simulink model "CraneStab"  (Simulink 8.6)
settings: Solver=ode1  SolverMode=SingleTasking  StartTime=0.0  StopTime=40  FixedStep=0.001  RelTol=1e-3
undefined symbols (not defined in the file): Advantech, PCI
libraries: sldrtlib x11
settings Model: Creator=Demo11  LastModifiedBy=demo  SimulationMode=external  ExtModeTrigMode=oneshot  ExtModeTrigDuration=100000
settings DataIOCC: LimitDataPoints=off  SignalLoggingName=sigsOut
settings OptimizationCC: BlockReduction=off  BooleanDataType=off  InitFltsAndDblsToZero=on
settings DebuggingCC: SaveWithParameterizedLinksMsg=none  SignalResolutionControl=TryResolveAllWithWarning  SolverPrmCheckMsg=none  MultiTaskDSMMsg=warning  MultiTaskCondExecSysMsg=none  FcnCallInpInsideContextMsg=UseLocalSettings
settings HardwareCC: ProdBitPerLong=64  ProdBitPerPointer=64  ProdIntDivRoundTo=Zero  ProdEndianess=LittleEndian  ProdWordSize=64  ProdHWDeviceType=Intel->x86-64  TargetBitPerLong=64  TargetBitPerPointer=64  TargetIntDivRoundTo=Zero  TargetEndianess=LittleEndian  TargetWordSize=64  TargetHWDeviceType=Intel->x86-64
settings RTWCC: SystemTargetFile=sldrt.tlc  TemplateMakefile=sldrt.tmf  Description=Simulink Desktop Real-Time  RTWCompilerOptimization=on
settings CodeAppCC: MaxIdLength=95
settings SimulinkDesktopRealTimeCC: TargetPreCompLibLocation=C:\Program Files\MATLAB\R2015b\toolbox\sldrt\lib\win64  TargetLangStandard=C89/C90 (ANSI)  SupportVariableSizeSignals=off

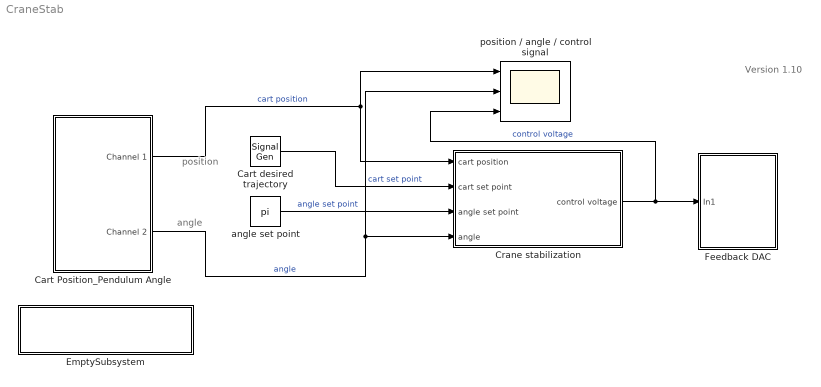
== system CraneStab ==
  note: position
  note: angle
  note: Version 1.10
  Cart Position_Pendulum Angle : Subsystem  mask(Feedback Encoder Block){st=0.001, of1=0, of2=-1024}
      mask prompts: st "Sample Time"; of1 "Channel 1 Offset"; of2 "Channel 2 Offset"
      mask help: Special block to use with the Feedback experiments to read encoder channels using the digital I/O lines
      mask Display:
      | image(imread('bckg.bmp'))
      | disp('PCI1711 \n Lab I/O Board \n\n\n Feedback Encoder')
  "Cart desired trajectory " : SignalGenerator  Amplitude=0.3  Frequency=0.1
  Crane stabilization : Subsystem
      mask Display:
      | image(imread('bckg.bmp'))
      | disp('Crane stabilization')
  EmptySubsystem : Subsystem
      mask Display:
      | image(imread('FB-inst-blue2.jpg'))
      | disp('\n\nFeedback Instruments Limited')
  Feedback DAC : Subsystem  mask(DAC Unit for Feedback Experiments){st=0.001, ch=1}
      mask prompts: st "Sample Time"; ch "Output Channel"
      mask help:
      | Digital to Analog Output  for Feedback Experiments
      | using Advantech PCI1711  I/O board
      mask Display:
      | image(imread('bckg.bmp'))
      | disp('PCI1711 \n Lab I/O Board \n\n Feedback  DAC')
  angle set point : Constant  Value=pi
  position / angle / control signal : Scope  NumInputPorts=3
      mask Display: image(imread('scope.jpg'))
  wires:
  Crane stabilization/1(control voltage) -> Feedback DAC/1(In1), position / angle / control signal/3  "control voltage"
  angle set point/1 -> Crane stabilization/3(angle set point)  "angle set point"
  Cart Position_Pendulum Angle/2(Channel 2) -> Crane stabilization/4(angle), position / angle / control signal/2  "angle"
  Cart Position_Pendulum Angle/1(Channel 1) -> Crane stabilization/1(cart position), position / angle / control signal/1  "cart position"
  "Cart desired trajectory "/1 -> Crane stabilization/2(cart set point)  "cart set point"

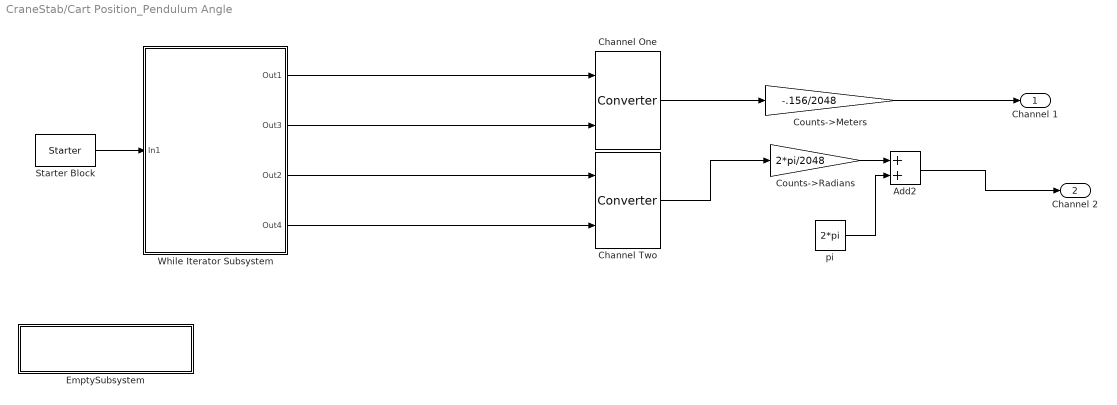
== system CraneStab/Cart Position_Pendulum Angle ==
  Add2 : Sum
  Channel One : S-Function  FunctionName=Converter  Parameters=of1,st  SFunctionDeploymentMode=off  EnableBusSupport=off
  Channel Two : S-Function  FunctionName=Converter  Parameters=of2,st  SFunctionDeploymentMode=off  EnableBusSupport=off
  Counts->Meters : Gain  Gain=-.156/2048  SaturateOnIntegerOverflow=on  OutDataTypeStr=Inherit: Same as input  ParamDataTypeStr=Inherit: Same as input
  Counts->Radians : Gain  Gain=2*pi/2048  SaturateOnIntegerOverflow=on  OutDataTypeStr=Inherit: Same as input  ParamDataTypeStr=Inherit: Same as input
  EmptySubsystem : Subsystem
      mask Display:
      | image(imread('FB-inst-blue2.jpg'))
      | disp('\n\nFeedback Instruments Limited')
  Starter Block : S-Function  FunctionName=Starter  Parameters=sample_time  SFunctionDeploymentMode=off  EnableBusSupport=off  mask{sample_time=st}
      mask prompts: sample_time "Sample Time:"
  While Iterator Subsystem : Subsystem  TreatAsAtomicUnit=on
  pi : Constant  Value=2*pi
  Channel 1 : Outport
  Channel 2 : Outport  Port=2
  wires:
  Add2/1 -> Channel 2/1
  Channel Two/1 -> Counts->Radians/1
  pi/1 -> Add2/2
  Counts->Radians/1 -> Add2/1
  Counts->Meters/1 -> Channel 1/1
  Starter Block/1 -> While Iterator Subsystem/1(In1)
  While Iterator Subsystem/1(Out1) -> Channel One/1
  While Iterator Subsystem/2(Out3) -> Channel One/2
  While Iterator Subsystem/3(Out2) -> Channel Two/1
  While Iterator Subsystem/4(Out4) -> Channel Two/2
  Channel One/1 -> Counts->Meters/1

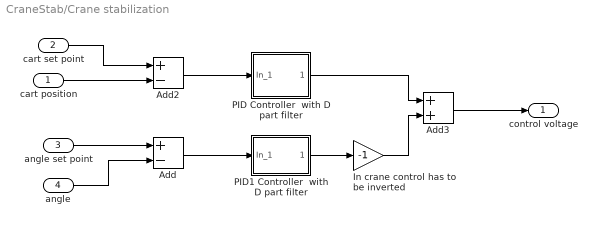
== system CraneStab/Crane stabilization ==
  cart position : Inport
  cart set point : Inport  Port=2
  angle set point : Inport  Port=3
  angle : Inport  Port=4
  Add : Sum  Inputs=+-
  Add2 : Sum  Inputs=+-
  Add3 : Sum
  In crane control has to be inverted : Gain  Gain=-1
  PID Controller  with D part filter : Subsystem  AncestorBlock=simulink_extras/Additional Linear/PID Controller  mask(PID Controller){P=8, I=0.3, D=4}
      mask prompts: P "Proportional:"; I "Integral:"; D "Derivative:"
      mask help:
      | Enter expressions for proportional, integral, and derivative terms.
      | P+I/s+Ds
      mask Help: This block implements a PID controller where parameters are entered for the Proportional, Integral and Derivative terms. Unmask this block to see how it works. The derivative term is implemented using a true derivative block.
      mask Callback P:
      | if str2num(get_param(gcb, 'P'))>12
      |  WARNDLG('Proportional Gain is out of the range [4..12] and is set to maximum value now', 'Setting Value Error')
      |  set_param(gcb,'P','12');
      | end
      | if str2num(get_param(gcb, 'P'))<4
      |  WARNDLG('Proportional Gain is out of the range [4..12] and is set to minimum now', 'Setting Value Error')
      |  set_param(gcb,'P','4');
      | end
      mask Callback I:
      | if str2num(get_param(gcb, 'I'))>0.5
      |  WARNDLG('Integral Gain is out of the range [0.1 .. 0.5] and is set to maximum value now', 'Setting Value Error')
      |  set_param(gcb,'I','0.5');
      | end
      | if str2num(get_param(gcb, 'I'))<0.1
      |  WARNDLG('Integral Gain is out of the range [0.1 .. 0.5] and is set to minimum now', 'Setting Value Error')
      |  set_param(gcb,'I','0.1');
      | end
      mask Callback D:
      | if str2num(get_param(gcb, 'D'))>6
      |  WARNDLG('Derivative Gain is out of the range [2..6] and is set to maximum value now', 'Setting Value Error')
      |  set_param(gcb,'D','6');
      | end
      | if str2num(get_param(gcb, 'D'))<2
      |  WARNDLG('Derivative Gain is out of the range [2..6] and is set to minimum now', 'Setting Value Error')
      |  set_param(gcb,'D','2');
      | end
      mask Display:
      | image(imread('bckg.bmp'))
      | disp('PID')
  PID1 Controller  with D part filter : Subsystem  AncestorBlock=simulink_extras/Additional Linear/PID Controller  mask(PID Controller){P=5, I=0.1, D=0.2}
      mask prompts: P "Proportional:"; I "Integral:"; D "Derivative:"
      mask help:
      | Enter expressions for proportional, integral, and derivative terms.
      | P+I/s+Ds
      mask Help: This block implements a PID controller where parameters are entered for the Proportional, Integral and Derivative terms. Unmask this block to see how it works. The derivative term is implemented using a true derivative block.
      mask Callback P:
      | if str2num(get_param(gcb, 'P'))>8
      |  WARNDLG('Proportional Gain is out of the range [2..8] and is set to maximum value now', 'Setting Value Error')
      |  set_param(gcb,'P','8');
      | end
      | if str2num(get_param(gcb, 'P'))<2
      |  WARNDLG('Proportional Gain is out of the range [2..8] and is set to minimum now', 'Setting Value Error')
      |  set_param(gcb,'P','2');
      | end
      mask Callback I:
      | if str2num(get_param(gcb, 'I'))>0.15
      |  WARNDLG('Integral Gain is out of the range [0.05 .. 0.15] and is set to maximum value now', 'Setting Value Error')
      |  set_param(gcb,'I','0.15');
      | end
      | if str2num(get_param(gcb, 'I'))<0.05
      |  WARNDLG('Integral Gain is out of the range [0.05 .. 0.15] and is set to minimum now', 'Setting Value Error')
      |  set_param(gcb,'I','0.05');
      | end
      mask Callback D:
      | if str2num(get_param(gcb, 'D'))>0.3
      |  WARNDLG('Derivative Gain is out of the range [0.1 .. 0.3] and is set to maximum value now', 'Setting Value Error')
      |  set_param(gcb,'D','0.3');
      | end
      | if str2num(get_param(gcb, 'D'))<0.1
      |  WARNDLG('Derivative Gain is out of the range [0.1 .. 0.3] and is set to minimum now', 'Setting Value Error')
      |  set_param(gcb,'D','0.1');
      | end
      mask Display:
      | image(imread('bckg.bmp'))
      | disp('PID')
  control voltage : Outport
  wires:
  angle/1 -> Add/2
  angle set point/1 -> Add/1
  cart set point/1 -> Add2/1
  cart position/1 -> Add2/2
  Add3/1 -> control voltage/1
  PID Controller  with D part filter/1(Out_1) -> Add3/1
  Add2/1 -> PID Controller  with D part filter/1(In_1)
  Add/1 -> PID1 Controller  with D part filter/1(In_1)
  In crane control has to be inverted/1 -> Add3/2
  PID1 Controller  with D part filter/1(Out_1) -> In crane control has to be inverted/1

== system CraneStab/EmptySubsystem ==

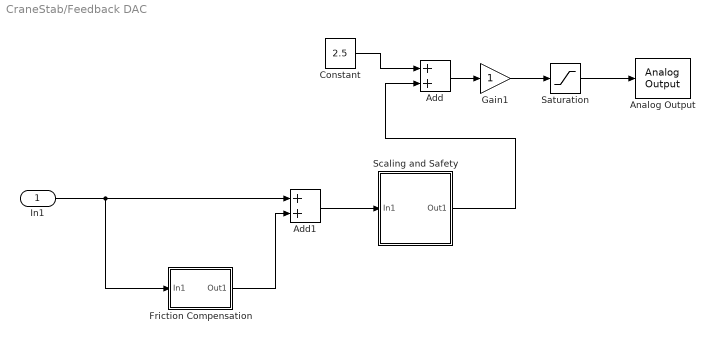
== system CraneStab/Feedback DAC ==
  In1 : Inport
  Add : Sum  OutDataTypeStr=Inherit: Same as first input
  Add1 : Sum
  Analog Output : sldrtlib/Analog Output  SampleTime=st  MaxMissedTicks=10  ShowMissedTicks=off  YieldWhenWaiting=off  DrvName=Advantech/PCI-1711  DrvAddress=4294967295  DrvOptions=zeros(1,0)  Channels=ch  RangeMode=1  VoltRange=2  InitialValue=2.5  FinalValue=2.5
      settings: AttributesFormatString=Advantech\nPCI-1711 [auto]
  Constant : Constant  Value=2.5
  Friction Compensation : Subsystem  mask(linear){frictionCompNeg=.1, frictionCompPos=.1}
      mask prompts: frictionCompNeg "Friction Compensation Magnitude in Negative Direction"; frictionCompPos "Friction Compensation Magnitude in Positive Direction"
      mask Display: plot(0,0,100,100,[40,30,20],[87,85,80],[46,54,54,46,46],[90,90,80,80,90],[46,45,45,46,54,55,55,54,46],[78,80,90,91,91,90,80,78,78],[51,51,49,49],[78,10,10,78],[90,80,70,60],[70,80,85,88],[20,10],[80,70],[20,20,15],[73,80,80],[85,80,80],[80,80,74])
  Gain1 : Gain
  Saturation : Saturate  UpperLimit=5.0  LowerLimit=0
  Scaling and Safety : Subsystem
  wires:
  Add1/1 -> Scaling and Safety/1(In1)
  In1/1 -> Add1/1, Friction Compensation/1(In1)
  Friction Compensation/1(Out1) -> Add1/2
  Constant/1 -> Add/1
  Saturation/1 -> Analog Output/1
  Add/1 -> Gain1/1
  Gain1/1 -> Saturation/1
  Scaling and Safety/1(Out1) -> Add/2

== system CraneStab/Cart Position_Pendulum Angle/EmptySubsystem ==

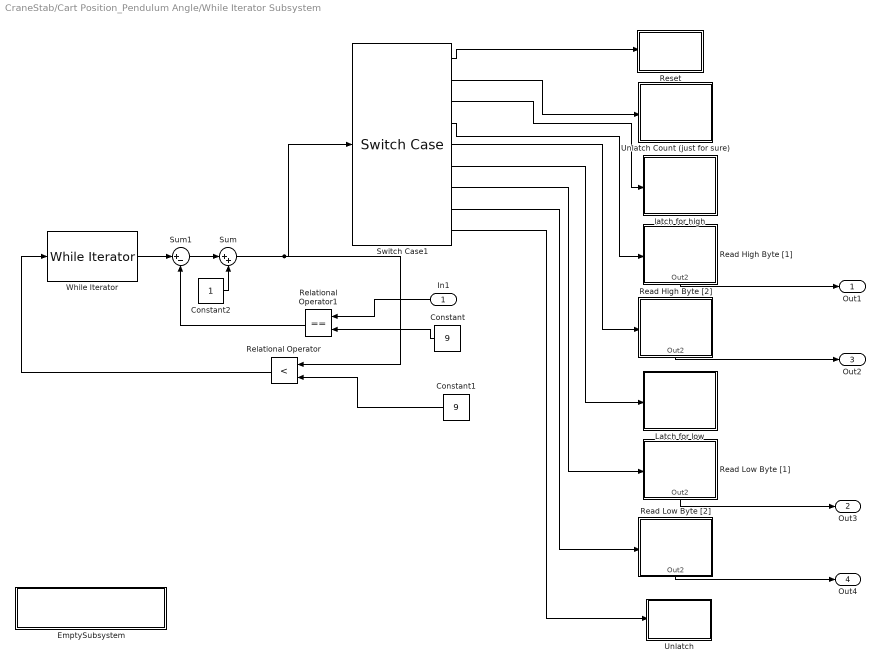
== system CraneStab/Cart Position_Pendulum Angle/While Iterator Subsystem ==
  In1 : Inport
  Constant : Constant  Value=9
  Constant1 : Constant  Value=9
  Constant2 : Constant
  EmptySubsystem : Subsystem
      mask Display:
      | image(imread('FB-inst-blue2.jpg'))
      | disp('\n\nFeedback Instruments Limited')
  Latch for low : Subsystem  TreatAsAtomicUnit=on
  Read High Byte [1] : Subsystem  TreatAsAtomicUnit=on
  Read High Byte [2] : Subsystem  TreatAsAtomicUnit=on
  Read Low Byte [1] : Subsystem  TreatAsAtomicUnit=on
  Read Low Byte [2] : Subsystem  TreatAsAtomicUnit=on
  Relational Operator : RelationalOperator  Operator=<  OutDataTypeStr=boolean
  Relational Operator1 : RelationalOperator  Operator===  OutDataTypeStr=boolean
  Reset : Subsystem  TreatAsAtomicUnit=on
  Sum : Sum  Inputs=|++
  Sum1 : Sum  Inputs=|+-  OutDataTypeStr=Inherit: Same as first input
  Switch Case1 : SwitchCase  CaseConditions={1,2,3,4,5,6,7,8,9}  ShowDefaultCase=off
  Unlatch : Subsystem  TreatAsAtomicUnit=on
  "Unlatch Count (just for sure) " : Subsystem  TreatAsAtomicUnit=on
  While Iterator : WhileIterator  MaxIters=9  WhileBlockType=do-while  ResetStates=reset  ShowIterationPort=on  OutputDataType=int8
  latch for high : Subsystem  TreatAsAtomicUnit=on
  Out1 : Outport
  Out3 : Outport  Port=2
  Out2 : Outport  Port=3
  Out4 : Outport  Port=4
  wires:
  Relational Operator/1 -> While Iterator/1
  In1/1 -> Relational Operator1/1
  Constant/1 -> Relational Operator1/2
  Relational Operator1/1 -> Sum1/2
  While Iterator/1 -> Sum1/1
  Switch Case1/1 -> Reset/Action
  Switch Case1/2 -> "Unlatch Count (just for sure) "/Action
  Constant1/1 -> Relational Operator/2
  Read High Byte [1]/1(Out2) -> Out1/1
  Read High Byte [2]/1(Out2) -> Out2/1
  Read Low Byte [1]/1(Out2) -> Out3/1
  Read Low Byte [2]/1(Out2) -> Out4/1
  Sum1/1 -> Sum/1
  Sum/1 -> Switch Case1/1, Relational Operator/1
  Constant2/1 -> Sum/2
  Switch Case1/3 -> latch for high/Action
  Switch Case1/4 -> Read High Byte [1]/Action
  Switch Case1/5 -> Read High Byte [2]/Action
  Switch Case1/6 -> Latch for low/Action
  Switch Case1/7 -> Read Low Byte [1]/Action
  Switch Case1/8 -> Read Low Byte [2]/Action
  Switch Case1/9 -> Unlatch/Action

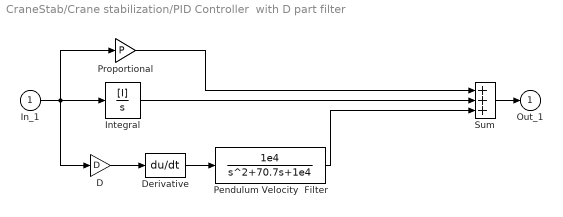
== system CraneStab/Crane stabilization/PID Controller  with D part filter ==
  In_1 : Inport
  D : Gain  Gain=D  SaturateOnIntegerOverflow=on  OutDataTypeStr=Inherit: Same as input  ParamDataTypeStr=Inherit: Same as input
  Derivative : Derivative
  Integral : TransferFcn  Numerator=[I]  Denominator=[1 0]
  Pendulum Velocity  Filter : TransferFcn  Numerator=[1e4]  Denominator=[1 70.7 1e4]
  Proportional : Gain  Gain=P  SaturateOnIntegerOverflow=on  OutDataTypeStr=Inherit: Same as input  ParamDataTypeStr=Inherit: Same as input
  Sum : Sum  Inputs=+++  SaturateOnIntegerOverflow=on  InputSameDT=on  OutDataTypeStr=Inherit: Same as first input
  Out_1 : Outport  InitialOutput=0
  wires:
  Pendulum Velocity  Filter/1 -> Sum/3
  D/1 -> Derivative/1
  Sum/1 -> Out_1/1
  In_1/1 -> Proportional/1, Integral/1, D/1
  Derivative/1 -> Pendulum Velocity  Filter/1
  Integral/1 -> Sum/2
  Proportional/1 -> Sum/1

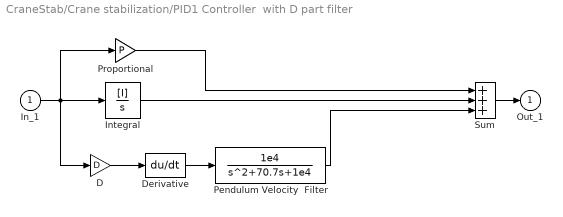
== system CraneStab/Crane stabilization/PID1 Controller  with D part filter ==
  In_1 : Inport
  D : Gain  Gain=D  SaturateOnIntegerOverflow=on  OutDataTypeStr=Inherit: Same as input  ParamDataTypeStr=Inherit: Same as input
  Derivative : Derivative
  Integral : TransferFcn  Numerator=[I]  Denominator=[1 0]
  Pendulum Velocity  Filter : TransferFcn  Numerator=[1e4]  Denominator=[1 70.7 1e4]
  Proportional : Gain  Gain=P  SaturateOnIntegerOverflow=on  OutDataTypeStr=Inherit: Same as input  ParamDataTypeStr=Inherit: Same as input
  Sum : Sum  Inputs=+++  SaturateOnIntegerOverflow=on  InputSameDT=on  OutDataTypeStr=Inherit: Same as first input
  Out_1 : Outport  InitialOutput=0
  wires:
  Proportional/1 -> Sum/1
  Integral/1 -> Sum/2
  Derivative/1 -> Pendulum Velocity  Filter/1
  In_1/1 -> Integral/1, Proportional/1, D/1
  Sum/1 -> Out_1/1
  D/1 -> Derivative/1
  Pendulum Velocity  Filter/1 -> Sum/3

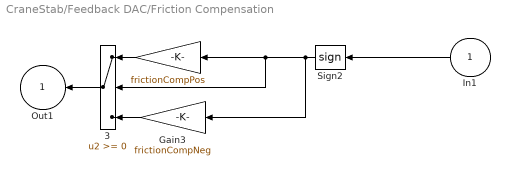
== system CraneStab/Feedback DAC/Friction Compensation ==
  In1 : Inport
  " " : Gain  Gain=frictionCompPos  SaturateOnIntegerOverflow=on  OutDataTypeStr=Inherit: Same as input  ParamDataTypeStr=Inherit: Same as input
  3 : Switch  SaturateOnIntegerOverflow=on  InputSameDT=on
  Gain3 : Gain  Gain=frictionCompNeg  SaturateOnIntegerOverflow=on  OutDataTypeStr=Inherit: Same as input  ParamDataTypeStr=Inherit: Same as input
  Sign2 : Signum  Tag=T
  Out1 : Outport  InitialOutput=0
  wires:
  3/1 -> Out1/1
  Sign2/1 -> 3/2, " "/1, Gain3/1
  Gain3/1 -> 3/3
  " "/1 -> 3/1
  In1/1 -> Sign2/1

== system CraneStab/Feedback DAC/Scaling and Safety ==
  In1 : Inport
  -1 : Gain  Gain=-1  SaturateOnIntegerOverflow=on  OutDataTypeStr=Inherit: Same as input  ParamDataTypeStr=Inherit: Same as input
  Saturation : Saturate  UpperLimit=2.5  LowerLimit=-2.5
  Out1 : Outport
  wires:
  -1/1 -> Saturation/1  "actual LoadPosition"
  In1/1 -> -1/1
  Saturation/1 -> Out1/1

== system CraneStab/Cart Position_Pendulum Angle/While Iterator Subsystem/EmptySubsystem ==

== system CraneStab/Cart Position_Pendulum Angle/While Iterator Subsystem/Latch for low ==
  Action Port : ActionPort  ActionType=case
  Constant : Constant  Value=6  OutDataTypeStr=double
  Digital Output : sldrtlib/Digital Output  SampleTime=-1  MaxMissedTicks=10  ShowMissedTicks=off  YieldWhenWaiting=off  DrvName=Advantech/PCI-1711  DrvAddress=4294967295  DrvOptions=zeros(1,0)  Channels=1  BitMode=2  InitialValue=0  FinalValue=0
      settings: AttributesFormatString=Advantech\nPCI-1711 [auto]
  wires:
  Constant/1 -> Digital Output/1

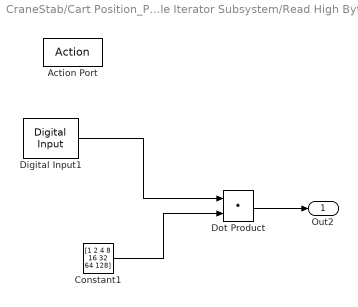
== system CraneStab/Cart Position_Pendulum Angle/While Iterator Subsystem/Read High Byte [1] ==
  Action Port : ActionPort  ActionType=case
  Constant1 : Constant  Value=[1 2 4 8 16 32 64 128]
  Digital Input1 : sldrtlib/Digital Input  SampleTime=-1  MaxMissedTicks=10  ShowMissedTicks=off  YieldWhenWaiting=off  DrvName=Advantech/PCI-1711  DrvAddress=4294967295  DrvOptions=zeros(1,0)  Channels=[1,2,3,4,5,6,7,8]  BitMode=1  DataType=1
      settings: AttributesFormatString=Advantech\nPCI-1711 [auto]
  Dot Product : DotProduct  InputSameDT=on  OutDataTypeStr=Inherit: Inherit via internal rule
  Out2 : Outport
  wires:
  Dot Product/1 -> Out2/1
  Constant1/1 -> Dot Product/2
  Digital Input1/1 -> Dot Product/1

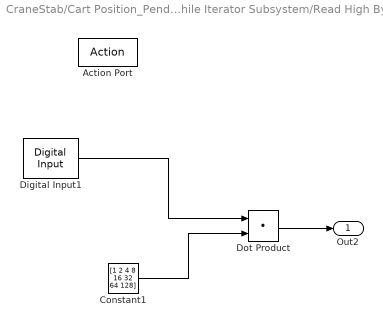
== system CraneStab/Cart Position_Pendulum Angle/While Iterator Subsystem/Read High Byte [2] ==
  Action Port : ActionPort  ActionType=case
  Constant1 : Constant  Value=[1 2 4 8 16 32 64 128]
  Digital Input1 : sldrtlib/Digital Input  SampleTime=-1  MaxMissedTicks=10  ShowMissedTicks=off  YieldWhenWaiting=off  DrvName=Advantech/PCI-1711  DrvAddress=4294967295  DrvOptions=zeros(1,0)  Channels=[9:16]  BitMode=1  DataType=1
      settings: AttributesFormatString=Advantech\nPCI-1711 [auto]
  Dot Product : DotProduct  InputSameDT=on  OutDataTypeStr=Inherit: Inherit via internal rule
  Out2 : Outport
  wires:
  Digital Input1/1 -> Dot Product/1
  Constant1/1 -> Dot Product/2
  Dot Product/1 -> Out2/1

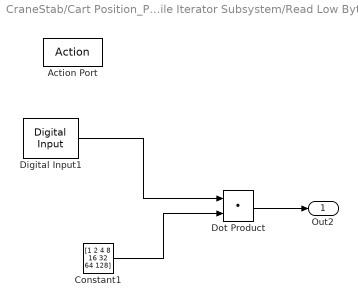
== system CraneStab/Cart Position_Pendulum Angle/While Iterator Subsystem/Read Low Byte [1] ==
  Action Port : ActionPort  ActionType=case
  Constant1 : Constant  Value=[1 2 4 8 16 32 64 128]
  Digital Input1 : sldrtlib/Digital Input  SampleTime=-1  MaxMissedTicks=10  ShowMissedTicks=off  YieldWhenWaiting=off  DrvName=Advantech/PCI-1711  DrvAddress=4294967295  DrvOptions=zeros(1,0)  Channels=[1:8]  BitMode=1  DataType=1
      settings: AttributesFormatString=Advantech\nPCI-1711 [auto]
  Dot Product : DotProduct  InputSameDT=on  OutDataTypeStr=Inherit: Inherit via internal rule
  Out2 : Outport
  wires:
  Digital Input1/1 -> Dot Product/1
  Constant1/1 -> Dot Product/2
  Dot Product/1 -> Out2/1

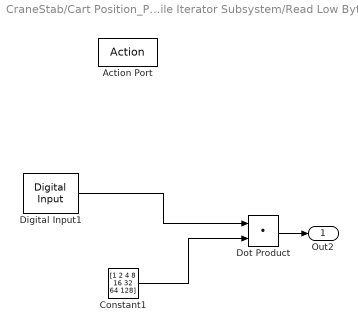
== system CraneStab/Cart Position_Pendulum Angle/While Iterator Subsystem/Read Low Byte [2] ==
  Action Port : ActionPort  ActionType=case
  Constant1 : Constant  Value=[1 2 4 8 16 32 64 128]
  Digital Input1 : sldrtlib/Digital Input  SampleTime=-1  MaxMissedTicks=10  ShowMissedTicks=off  YieldWhenWaiting=off  DrvName=Advantech/PCI-1711  DrvAddress=4294967295  DrvOptions=zeros(1,0)  Channels=[9:16]  BitMode=1  DataType=1
      settings: AttributesFormatString=Advantech\nPCI-1711 [auto]
  Dot Product : DotProduct  InputSameDT=on  OutDataTypeStr=Inherit: Inherit via internal rule
  Out2 : Outport
  wires:
  Constant1/1 -> Dot Product/2
  Digital Input1/1 -> Dot Product/1
  Dot Product/1 -> Out2/1

== system CraneStab/Cart Position_Pendulum Angle/While Iterator Subsystem/Reset ==
  Action Port : ActionPort  ActionType=case
  Constant : Constant  Value=3  OutDataTypeStr=double
  Digital Output1 : sldrtlib/Digital Output  SampleTime=-1  MaxMissedTicks=10  ShowMissedTicks=off  YieldWhenWaiting=off  DrvName=Advantech/PCI-1711  DrvAddress=4294967295  DrvOptions=zeros(1,0)  Channels=1  BitMode=2  InitialValue=0  FinalValue=0
      settings: AttributesFormatString=Advantech\nPCI-1711 [auto]
  Subsystem : Subsystem
  wires:
  Constant/1 -> Subsystem/1(In1)
  Subsystem/1(Out1) -> Digital Output1/1

== system CraneStab/Cart Position_Pendulum Angle/While Iterator Subsystem/Unlatch ==
  Action Port : ActionPort  ActionType=case
  Constant : Constant  Value=7  OutDataTypeStr=double
  Digital Output1 : sldrtlib/Digital Output  SampleTime=-1  MaxMissedTicks=10  ShowMissedTicks=off  YieldWhenWaiting=off  DrvName=Advantech/PCI-1711  DrvAddress=4294967295  DrvOptions=zeros(1,0)  Channels=1  BitMode=2  InitialValue=0  FinalValue=0
      settings: AttributesFormatString=Advantech\nPCI-1711 [auto]
  wires:
  Constant/1 -> Digital Output1/1

== system CraneStab/Cart Position_Pendulum Angle/While Iterator Subsystem/Unlatch Count (just for sure)  ==
  Action Port : ActionPort  ActionType=case
  Constant : Constant  Value=7  OutDataTypeStr=double
  Digital Output : sldrtlib/Digital Output  SampleTime=-1  MaxMissedTicks=10  ShowMissedTicks=off  YieldWhenWaiting=off  DrvName=Advantech/PCI-1711  DrvAddress=4294967295  DrvOptions=zeros(1,0)  Channels=1  BitMode=2  InitialValue=0  FinalValue=0
      settings: AttributesFormatString=Advantech\nPCI-1711 [auto]
  wires:
  Constant/1 -> Digital Output/1

== system CraneStab/Cart Position_Pendulum Angle/While Iterator Subsystem/latch for high ==
  Action Port : ActionPort  ActionType=case
  Constant : Constant  Value=4  OutDataTypeStr=double
  Digital Output : sldrtlib/Digital Output  SampleTime=-1  MaxMissedTicks=10  ShowMissedTicks=off  YieldWhenWaiting=off  DrvName=Advantech/PCI-1711  DrvAddress=4294967295  DrvOptions=zeros(1,0)  Channels=1  BitMode=2  InitialValue=0  FinalValue=0
      settings: AttributesFormatString=Advantech\nPCI-1711 [auto]
  wires:
  Constant/1 -> Digital Output/1

== system CraneStab/Cart Position_Pendulum Angle/While Iterator Subsystem/Reset/Subsystem ==
  In1 : Inport
  Constant1 : Constant  Value=7  OutDataTypeStr=double
  Digital Output : sldrtlib/Digital Output  SampleTime=-1  MaxMissedTicks=10  ShowMissedTicks=off  YieldWhenWaiting=off  DrvName=Advantech/PCI-1711  DrvAddress=4294967295  DrvOptions=zeros(1,0)  Channels=[1 2 3]  BitMode=2  InitialValue=0  FinalValue=0
      settings: AttributesFormatString=Advantech\nPCI-1711 [auto]
  Out1 : Outport
  wires:
  Constant1/1 -> Out1/1
  In1/1 -> Digital Output/1
